simulink model "linear_control_scheme_22b"  (R2022b)
settings: Solver=VariableStepAuto  StartTime=0.0  StopTime=10.0  RelTol=1e-3
InitFcn:
  | init_linear
undefined symbols (not defined in the file or in its folder): pa
settings Model: Creator=HQ03  LastModifiedBy=HQ03

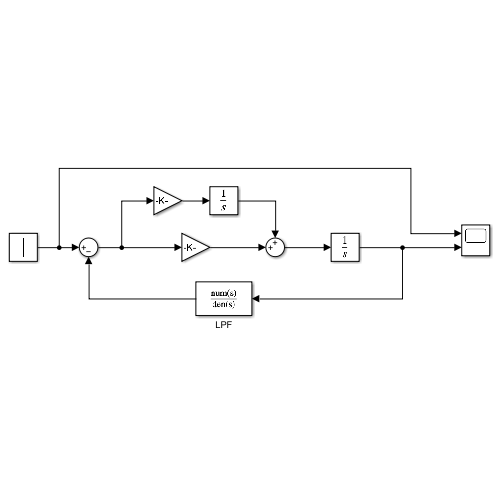
[thumbnail: Simulink's stored preview of the top-level diagram]
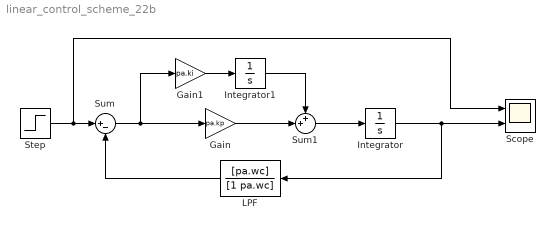
== system linear_control_scheme_22b ==
  Gain : Gain  Gain=pa.kp
  Gain1 : Gain  Gain=pa.ki
  Integrator : Integrator
  Integrator1 : Integrator
  LPF : TransferFcn  Numerator=[pa.wc]  Denominator=[1 pa.wc]
  Scope : Scope  NumInputPorts=2
  Step : Step  SampleTime=0
  Sum : Sum  Inputs=|+-
  Sum1 : Sum  Inputs=++|
  wires:
  Sum/1 -> Gain1/1, Gain/1
  Integrator/1 -> LPF/1, Scope/2
  Gain1/1 -> Integrator1/1
  Sum1/1 -> Integrator/1
  Gain/1 -> Sum1/2
  Integrator1/1 -> Sum1/1
  LPF/1 -> Sum/2
  Step/1 -> Scope/1, Sum/1
